simulink model "PI_kalman_discreto"  (R2023b)
settings: Solver=VariableStepAuto  StartTime=0.0  StopTime=200  RelTol=1e-3
undefined symbols (not defined in the file): C_ss, CI, DI, Discrete, dVdt, Ki1, Ki2, Kp1, Kp2, Rn, sigma, step_temp, steptime, Time, Ts, Tsp, Ufeedforward, V0, Vb0, Vmax, Vmin, wd
libraries: slpidlib x2, ctrlSharedLib x1, simulink x1
settings Model: Creator=Maialen  LastModifiedBy=Maialen

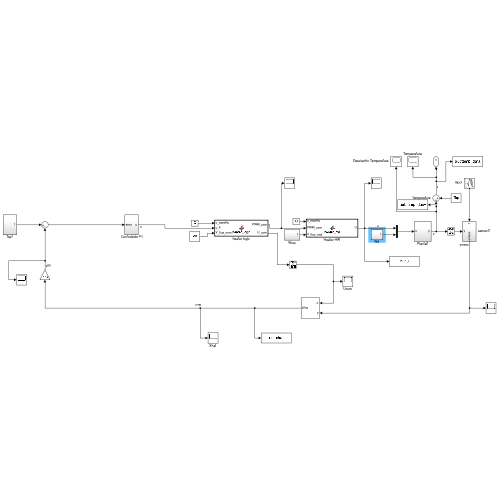
[thumbnail: Simulink's stored preview of the top-level diagram]
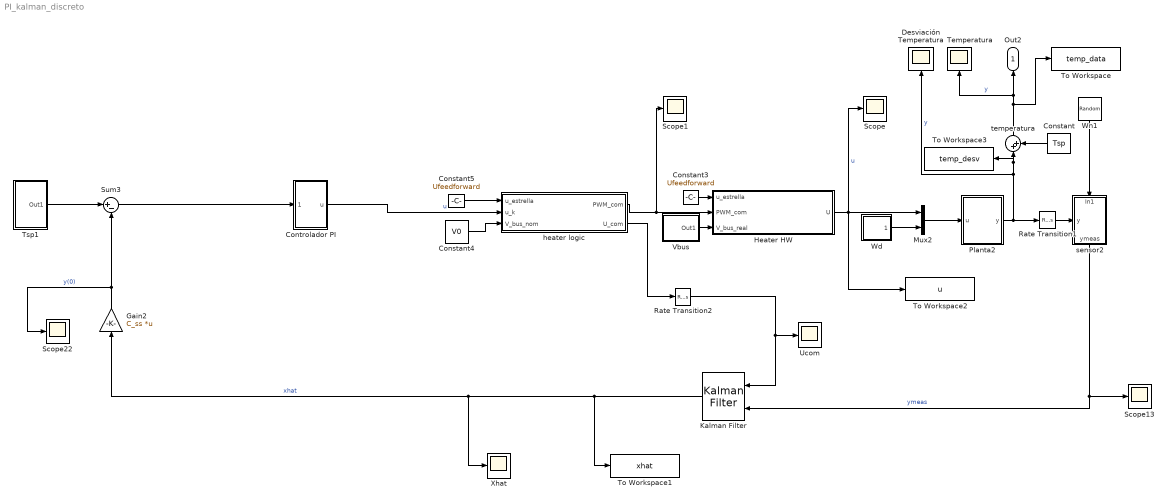
== system PI_kalman_discreto ==
  " Controlador PI" : Subsystem
  Constant : Constant  Value=Tsp  SampleTime=0
  Constant3 : Constant  Value=Ufeedforward  SampleTime=0
  Constant4 : Constant  Value=V0  SampleTime=0
  Constant5 : Constant  Value=Ufeedforward  SampleTime=0
  Desviación Temperatura : Scope
  Gain2 : Gain  Gain=C_ss  Multiplication=Matrix(K*u)
  Heater HW : MATLAB Function  TreatAsAtomicUnit=on
  Kalman Filter : ctrlSharedLib/Kalman Filter  TimeDomain=Discrete-Time  UseCurrentEstimator=on  ModelSource=LTI State-Space Variable  ModelSourceVariable=syskf  A=0.95  B=1  C=1  D=0  NumberOfStates=1  NumberOfInputs=1  NumberOfOutputs=1  InitialEstimateSource=Dialog  X0=0  P0=10  UseK=off  UseGH=off  NumberOfProcessNoiseInputs=1  G=1  TimeInvariantG=on  H=0  TimeInvariantH=on  Q=Qn  TimeInvariantQ=on  R=Rn  TimeInvariantR=on  N=0  TimeInvariantN=on  AddInputPort=on  AddEnablePort=off  OutputEstimatedY=off  OutputP=off  Ts=-1
  Mux2 : Mux  Inputs=2
  Planta2 : Subsystem
  Rate Transition1 : RateTransition  OutPortSampleTime=Ts
  Rate Transition2 : RateTransition  OutPortSampleTime=Ts
  Scope{,1,13,22} (4 alike) : Scope
  Sum3 : Sum  Inputs=|+-
  Temperatura : Scope
  To Workspace : ToWorkspace  VariableName=temp_data  SaveFormat=Timeseries  SampleTime=-1
  To Workspace1 : ToWorkspace  VariableName=xhat  SaveFormat=Timeseries  SampleTime=-1
  To Workspace2 : ToWorkspace  VariableName=u  SaveFormat=Timeseries  SampleTime=-1
  To Workspace3 : ToWorkspace  VariableName=temp_desv  SaveFormat=Timeseries  SampleTime=-1
  Tsp1 : Subsystem
  Ucom : Scope
  Vbus : Subsystem
  Wd : Subsystem
  Wn1 : RandomNumber  Variance=sigma^2  SampleTime=Ts
  Xhat : Scope
  heater logic : MATLAB Function  TreatAsAtomicUnit=on
  sensor2 : Subsystem
      settings: PortSchema="{\"entries\":[{\"content\":{\"sides\":[{\"content\":{\"connectorIds\":[\"In1\"]},\"type\":\"ConnectorPlacement.EquallySpacedRectSide\",\"uuid\":\"87c57665-5a3a-4a29-be31-fc3b8356ea98\"},{\"content\":{\"connectorIds\":[\"Out1\"],\"side\":\"RIGHT\"},\"type\":\"ConnectorPlacement.EquallySpacedRectSide\",\"uuid\":\"3fe956b0-7f9e-4b46-bcb6-e49be4c7e683\"},{\"content\":{\"connectorIds\":[\"In2\"],\"side\":\"TOP\"},\"type\":\"ConnectorPlacement.EquallySpacedRectSide\",\"uuid\":\"3d207620-bc84-4c0d-9751-3dea453ac424\"}]},\"type\":\"ConnectorPlacement.EquallySpacedConnector\",\"uuid\":\"7e1a59fd-e04d-40d6-8549-9ebaaabea5d7\"}],\"packageUris\":[\"http://schema.mathworks.com/mf0/Connector/R2020b\"],\"version\":\"1.0\"}"
  temperatura : Sum  Inputs=|++
  Out2 : Outport
  wires:
  Vbus/1(Out1) -> Heater HW/3(V_bus_real)
  Planta2/1(y) -> Desviación Temperatura/1, To Workspace3/1, temperatura/1, Rate Transition1/1  "y"
  sensor2/1(ymeas) -> Kalman Filter/2, Scope13/1  "ymeas"
  Gain2/1 -> Sum3/2, Scope22/1  "y(0)"
  Wd/1(Out1) -> Mux2/2
  Constant/1 -> temperatura/2
  Constant5/1 -> heater logic/1(u_estrella)
  Wn1/1 -> sensor2/1(In1)
  heater logic/1(PWM_com) -> Heater HW/2(PWM_com), Scope1/1
  Heater HW/1(U) -> Mux2/1, To Workspace2/1, Scope/1  "u"
  Constant4/1 -> heater logic/3(V_bus_nom)
  Constant3/1 -> Heater HW/1(u_estrella)
  Kalman Filter/1 -> To Workspace1/1, Gain2/1, Xhat/1  "xhat"
  Tsp1/1(Out1) -> Sum3/1
  Mux2/1 -> Planta2/1(u)
  temperatura/1 -> To Workspace/1, Temperatura/1, Out2/1  "y"
  heater logic/2(U_com) -> Rate Transition2/1
  Sum3/1 -> " Controlador PI"/1(error)
  " Controlador PI"/1(u) -> heater logic/2(u_k)  "u"
  Rate Transition1/1 -> sensor2/2(y)
  Rate Transition2/1 -> Ucom/1, Kalman Filter/1

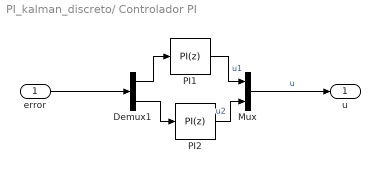
== system PI_kalman_discreto/ Controlador PI ==
  error : Inport
  Demux1 : Demux  Outputs=2
  Mux : Mux  Inputs=2
  "PI1 " : slpidlib/PID Controller  Controller=PI  Form=Parallel  TimeDomain=Discrete-time  UseExternalTs=off  SampleTime=Ts  IntegratorMethod=Forward Euler  FilterMethod=Forward Euler  ControllerParametersSource=internal  P=Kp1  I=Ki1  UseKiTs=off  D=0  N=100  UseFilter=on  TunerSelectOption=Transfer Function Based (PID Tuner App)  InitialConditionSource=internal  InitialConditionForIntegrator=0  InitialConditionForFilter=0  DifferentiatorICPrevScaledInput=0  ExternalReset=none  TrackingMode=off  Kt=1  LimitOutput=off  SatLimitsSource=internal  UpperSaturationLimit=5.7398  LowerSaturationLimit=-5.7398  LinearizeAsGain=on  AntiWindupMode=none  Kb=1  LimitIntegrator=on  UpperIntegratorSaturationLimit=P0  LowerIntegratorSaturationLimit=0  POutMin=[]  POutMax=[]  IOutMin=[]  IOutMax=[]  DOutMin=[]  DOutMax=[]  NOutMin=[]  NOutMax=[]  SumOutMin=[]  SumOutMax=[]  SaturationOutMin=[]  SaturationOutMax=[]  PParamMin=[]  PParamMax=[]  IParamMin=[]  IParamMax=[]  DParamMin=[]  DParamMax=[]  NParamMin=[]  NParamMax=[]  KbParamMin=[]  KbParamMax=[]  KtParamMin=[]  KtParamMax=[]  KbOutMin=[]  KbOutMax=[]  KtOutMin=[]  KtOutMax=[]  IntegratorOutMin=[]  IntegratorOutMax=[]  FilterOutMin=[]  FilterOutMax=[]  SumI1OutMin=[]  SumI1OutMax=[]  SumI2OutMin=[]  SumI2OutMax=[]  SumI3OutMin=[]  SumI3OutMax=[]  SumI4OutMin=[]  SumI4OutMax=[]  SumDOutMin=[]  SumDOutMax=[]  DifferentiatorOutMin=[]  DifferentiatorOutMax=[]  FilterDiffOutCoefMin=[]  FilterDiffOutCoefMax=[]  ReciprocalOutMin=[]  ReciprocalOutMax=[]  SumDenOutMin=[]  SumDenOutMax=[]  SumNumOutMin=[]  SumNumOutMax=[]  DivideOutMin=[]  DivideOutMax=[]  UdiffTsProdOutMin=[]  UdiffTsProdOutMax=[]  NTsProdOutMin=[]  NTsProdOutMax=[]  UintegralTsProdOutMin=[]  UintegralTsProdOutMax=[]  UngainTsProdOutMin=[]  UngainTsProdOutMax=[]  ClampingZeroOutDataTypeStr=Inherit: Inherit via back propagation  ClampingZeroOutMin=[]  ClampingZeroOutMax=[]  FilterDenConstantOutDataTypeStr=Inherit: Inherit via back propagation  FilterDenConstantOutMin=[]  FilterDenConstantOutMax=[]  PCopyOutDataTypeStr=Inherit: Inherit via back propagation  PCopyOutMin=[]  PCopyOutMax=[]  NCopyOutDataTypeStr=Inherit: Inherit via back propagation  NCopyOutMin=[]  NCopyOutMax=[]  IntegratorContinuousStateAttributes=''  IntegratorStateMustResolveToSignalObject=off  IntegratorRTWStateStorageClass=Auto  FilterContinuousStateAttributes=''  FilterStateMustResolveToSignalObject=off  FilterRTWStateStorageClass=Auto  ParallelPVariant=InternalParameters  IdealPVariant=Disabled  IVariant=InternalParameters  DVariant=Disabled  IntegratorVariant=Discrete  SatVariant=Disabled  AWVariant=Passthrough  PCopyVariant=Disabled  TRVariant=Disabled  FdbkBlocksVariant=Forward  IdealPFdbkVariant=Disabled  SatFdbkVariant=Disabled  DerivativeFilterVariant=Disabled  NVariant=Disabled  NCopyVariant=Disabled_SignalSpec  FilterICVariant=Disabled  IntegratorICVariant=InternalICs  ExternalResetVariant=Disabled  TRSumVariant=Passthrough  SumFdbkVariant=Disabled  SumVariant=Sum_PI  TsampFilterVariant=InternalTs  TsampNgainVariant=Passthrough  TsampIntegralVariant=Disabled_SignalSpec  ExternalSaturationOutDataTypeStr=Inherit: Same as second input
  "PI2 " : slpidlib/PID Controller  Controller=PI  Form=Parallel  TimeDomain=Discrete-time  UseExternalTs=off  SampleTime=Ts  IntegratorMethod=Forward Euler  FilterMethod=Forward Euler  ControllerParametersSource=internal  P=Kp2  I=Ki2  UseKiTs=off  D=0  N=100  UseFilter=on  TunerSelectOption=Transfer Function Based (PID Tuner App)  InitialConditionSource=internal  InitialConditionForIntegrator=0  InitialConditionForFilter=0  DifferentiatorICPrevScaledInput=0  ExternalReset=none  TrackingMode=off  Kt=1  LimitOutput=off  SatLimitsSource=internal  UpperSaturationLimit=5.7398  LowerSaturationLimit=-5.7398  LinearizeAsGain=on  AntiWindupMode=none  Kb=1  LimitIntegrator=on  UpperIntegratorSaturationLimit=P0  LowerIntegratorSaturationLimit=0  POutMin=[]  POutMax=[]  IOutMin=[]  IOutMax=[]  DOutMin=[]  DOutMax=[]  NOutMin=[]  NOutMax=[]  SumOutMin=[]  SumOutMax=[]  SaturationOutMin=[]  SaturationOutMax=[]  PParamMin=[]  PParamMax=[]  IParamMin=[]  IParamMax=[]  DParamMin=[]  DParamMax=[]  NParamMin=[]  NParamMax=[]  KbParamMin=[]  KbParamMax=[]  KtParamMin=[]  KtParamMax=[]  KbOutMin=[]  KbOutMax=[]  KtOutMin=[]  KtOutMax=[]  IntegratorOutMin=[]  IntegratorOutMax=[]  FilterOutMin=[]  FilterOutMax=[]  SumI1OutMin=[]  SumI1OutMax=[]  SumI2OutMin=[]  SumI2OutMax=[]  SumI3OutMin=[]  SumI3OutMax=[]  SumI4OutMin=[]  SumI4OutMax=[]  SumDOutMin=[]  SumDOutMax=[]  DifferentiatorOutMin=[]  DifferentiatorOutMax=[]  FilterDiffOutCoefMin=[]  FilterDiffOutCoefMax=[]  ReciprocalOutMin=[]  ReciprocalOutMax=[]  SumDenOutMin=[]  SumDenOutMax=[]  SumNumOutMin=[]  SumNumOutMax=[]  DivideOutMin=[]  DivideOutMax=[]  UdiffTsProdOutMin=[]  UdiffTsProdOutMax=[]  NTsProdOutMin=[]  NTsProdOutMax=[]  UintegralTsProdOutMin=[]  UintegralTsProdOutMax=[]  UngainTsProdOutMin=[]  UngainTsProdOutMax=[]  ClampingZeroOutDataTypeStr=Inherit: Inherit via back propagation  ClampingZeroOutMin=[]  ClampingZeroOutMax=[]  FilterDenConstantOutDataTypeStr=Inherit: Inherit via back propagation  FilterDenConstantOutMin=[]  FilterDenConstantOutMax=[]  PCopyOutDataTypeStr=Inherit: Inherit via back propagation  PCopyOutMin=[]  PCopyOutMax=[]  NCopyOutDataTypeStr=Inherit: Inherit via back propagation  NCopyOutMin=[]  NCopyOutMax=[]  IntegratorContinuousStateAttributes=''  IntegratorStateMustResolveToSignalObject=off  IntegratorRTWStateStorageClass=Auto  FilterContinuousStateAttributes=''  FilterStateMustResolveToSignalObject=off  FilterRTWStateStorageClass=Auto  ParallelPVariant=InternalParameters  IdealPVariant=Disabled  IVariant=InternalParameters  DVariant=Disabled  IntegratorVariant=Discrete  SatVariant=Disabled  AWVariant=Passthrough  PCopyVariant=Disabled  TRVariant=Disabled  FdbkBlocksVariant=Forward  IdealPFdbkVariant=Disabled  SatFdbkVariant=Disabled  DerivativeFilterVariant=Disabled  NVariant=Disabled  NCopyVariant=Disabled_SignalSpec  FilterICVariant=Disabled  IntegratorICVariant=InternalICs  ExternalResetVariant=Disabled  TRSumVariant=Passthrough  SumFdbkVariant=Disabled  SumVariant=Sum_PI  TsampFilterVariant=InternalTs  TsampNgainVariant=Passthrough  TsampIntegralVariant=Disabled_SignalSpec  ExternalSaturationOutDataTypeStr=Inherit: Same as second input
  u : Outport
  wires:
  Mux/1 -> u/1  "u"
  "PI1 "/1 -> Mux/1  "u1"
  error/1 -> Demux1/1
  Demux1/2 -> "PI2 "/1
  "PI2 "/1 -> Mux/2  "u2"
  Demux1/1 -> "PI1 "/1

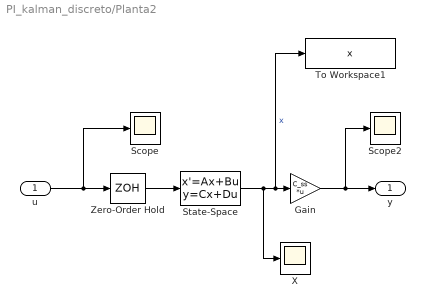
== system PI_kalman_discreto/Planta2 ==
  u : Inport
  Gain : Gain  Gain=C_ss  Multiplication=Matrix(K*u)
  Scope : Scope
  Scope2 : Scope
  State-Space : StateSpace  A=[-28.285755 18.000026 0 0 0 0 0 10.285729 0 0 0 0 0 0 0 0 0 0 0 0 0 0 0 0 0 0 0 0 0 0 0 0 0 0 0 0 0 0;18.000026 -36.000051 18.000026 0 0 0 0 0 0 0 0 0 0 0 0 0 0 0 0 0 0 0 0 0 0 0 0 0 0 0 0 0 0 0 0 0 0 0;0 18.000026 -28.285755 0 0 0 0 0 0 0 0 0 0 0 0 0 0 0 0 0 0 0 0 0 0 0 0 0 0 0 0 0 10.285729 0 0 0 0 0;0 0 0 -28.285755 18.000026 0 10.285729 0 0 0 0 0 0 0 0 0 0 0 0 0 0 0 0 0 0 0 0 0 0 0 0 0 0 0 0 0 0 0;0 0 0 18.000026 -36.000051 18.000026 0 0 0 0 0 0 0 0 0 0 0 0 0 0 0 0 0 0 0 0 0 0 0 0 0 0 0 0 0 0 0 0;0 0 0 0 18.000026 -28.285755 0 0 0 0 0 0 0 0 0 0 0 0 0 0 0 0 0 0 0 0 0 0 0 0 0 0 10.285729 0 0 0 0 0;0 0 0 48 0 0 -48 0 0 0 0 0 0 0 0 0 0 0 0 0 0 0 0 0 0 0 0 0 0 0 0 0 0 0 0 0 0 0;48 0 0 0 0 0 0 -48 0 0 0 0 0 0 0 0 0 0 0 0 0 0 0 0 0 0 0 0 0 0 0 0 0 0 0 0 0 0;0 0 0 0 0 0 0 0 -0.018321982 0.010128496 0 0 0 0 0.0081027967 0 0 0 0 0 0 0 0 0 0 0 0 0 0 0 0 0 0 0 0 0 0 0;0 0 0 0 0 0 0 0 0.010128496 -0.028450675 0.010128496 0 0 0 0 0.0081027967 0 0 0 0 0 0 0 0 0 0 0 0 0 0 0 0 0 0 0 0 0 0;0 0 0 0 0 0 0 0 0 0.010128496 -0.028450922 0.010128496 0 0 0 0 0.0081027967 0 0 0 0 0 0 0 0 0 0 0 0 0 0 0 0 0 0 0 0 0;0 0 0 0 0 0 0 0 0 0 0.010128496 -0.028450922 0.010128496 0 0 0 0 0.0081027967 0 0 0 0 0 0 0 0 0 0 0 0 0 0 0 0 0 0 0 0;0 0 0 0 0 0 0 0 0 0 0 0.010128496 -0.028450675 0.010128496 0 0 0 0 0.0081027967 0 0 0 0 0 0 0 0 0 0 0 0 0 0 0 0 0 0 0;0 0 0 0 0 0 0 0 0 0 0 0 0.010128496 -0.018321982 0 0 0 0 0 0.0081027967 0 0 0 0 0 0 0 0 0 0 0 0 0 0 0 0 0 0;0 0 0 0 0 0 0 0 0.0081027967 0 0 0 0 0 -0.026425101 0.010128496 0 0 0 0 0.0081027967 0 0 0 0 0 0 0 0 0 0 0 0 0 0 0 0 0;0 0 0 0 0 0 0 0 0 0.0081027967 0 0 0 0 0.010128496 -0.036553982 0.010128496 0 0 0 0 0.0081027967 0 0 0 0 0 0 0 0 0 0 0 0 0 0 0 0;0 0 0 0 0 0 0 0 0 0 0.0081027967 0 0 0 0 0.010128496 -0.036554604 0.010128496 0 0 0 0 0.0081027967 0 0 0 0 0 0 0 0 0 0 0 0 0 0 0;0 0 0 0 0 0 0 0 0 0 0 0.0081027967 0 0 0 0 0.010128496 -0.036554604 0.010128496 0 0 0 0 0.0081027967 0 0 0 0 0 0 0 0 0 0 0 0 0 0;0 0 0 0 0 0 0 0 0 0 0 0 0.0081027967 0 0 0 0 0.010128496 -0.036553982 0.010128496 0 0 0 0 0.0081027967 0 0 0 0 0 0 0 0 0 0 0 0 0;0 0 0 0 0 0 0 0 0 0 0 0 0 0.0081027967 0 0 0 0 0.010128496 -0.026425101 0 0 0 0 0 0.0081027967 0 0 0 0 0 0 0 0 0 0 0 0;0 0 0 0 0 0 0 0 0 0 0 0 0 0 0.0081027967 0 0 0 0 0 -0.026425515 0.010128496 0 0 0 0 0.0081027967 0 0 0 0 0 0 0 0 0 0 0;0 0 0 0 0 0 0 0 0 0 0 0 0 0 0 0.0081027967 0 0 0 0 0.010128496 -0.03655478 0.010128496 0 0 0 0 0.0081027967 0 0 0 0 0 0 0 0 0 0;0 0 0 0 0 0 0 0 0 0 0 0 0 0 0 0 0.0081027967 0 0 0 0 0.010128496 -0.089051211 0.010128496 0 0 0 0 0.0081027967 0 0 0 0 0 0 0 0 0.052494331;0 0 0 0 0 0 0 0 0 0 0 0 0 0 0 0 0 0.0081027967 0 0 0 0 0.010128496 -0.089051211 0.010128496 0 0 0 0 0.0081027967 0 0 0 0 0 0 0 0.052494331;0 0 0 0 0 0 0 0 0 0 0 0 0 0 0 0 0 0 0.0081027967 0 0 0 0 0.010128496 -0.03655478 0.010128496 0 0 0 0 0.0081027967 0 0 0 0 0 0 0;0 0 0 0 0 0 0 0 0 0 0 0 0 0 0 0 0 0 0 0.0081027967 0 0 0 0 0.010128496 -0.026425515 0 0 0 0 0 0.0081027967 0 0 0 0 0 0;0 0 0 0 0 0 0 0 0 0 0 0 0 0 0 0 0 0 0 0 0.0081027967 0 0 0 0 0 -0.018322752 0.010128496 0 0 0 0 0 0 0 0 0 0;0 0 0 0 0 0 0 0 0 0 0 0 0 0 0 0 0 0 0 0 0 0.0081027967 0 0 0 0 0.010128496 -0.028451741 0.010128496 0 0 0 0 0 0 0 0 0;0 0 0 0 0 0 0 0 0 0 0 0 0 0 0 0 0 0 0 0 0 0 0.0081027967 0 0 0 0 0.010128496 -0.02845251 0.010128496 0 0 0 0 0 0 0 0;0 0 0 0 0 0 0 0 0 0 0 0 0 0 0 0 0 0 0 0 0 0 0 0.0081027967 0 0 0 0 0.010128496 -0.02845251 0.010128496 0 0 0 0 0 0 0;0 0 0 0 0 0 0 0 0 0 0 0 0 0 0 0 0 0 0 0 0 0 0 0 0.0081027967 0 0 0 0 0.010128496 -0.028451741 0.010128496 0 0 0 0 0 0;0 0 0 0 0 0 0 0 0 0 0 0 0 0 0 0 0 0 0 0 0 0 0 0 0 0.0081027967 0 0 0 0 0.010128496 -0.018322752 0 0 0 0 0 0;0 0 2.2857143 0 0 2.2857143 0 0 0 0 0 0 0 0 0 0 0 0 0 0 0 0 0 0 0 0 0 0 0 0 0 0 -9.3428571 4.7714286 0 0 0 0;0 0 0 0 0 0 0 0 0 0 0 0 0 0 0 0 0 0 0 0 0 0 0 0 0 0 0 0 0 0 0 0 4.7714286 -9.5428571 4.7714286 0 0 0;0 0 0 0 0 0 0 0 0 0 0 0 0 0 0 0 0 0 0 0 0 0 0 0 0 0 0 0 0 0 0 0 0 4.7714286 -10.228571 5.4571429 0 0;0 0 0 0 0 0 0 0 0 0 0 0 0 0 0 0 0 0 0 0 0 0 0 0 0 0 0 0 0 0 0 0 0 0 5.4571429 -11.819048 6.3619048 0;0 0 0 0 0 0 0 0 0 0 0 0 0 0 0 0 0 0 0 0 0 0 0 0 0 0 0 0 0 0 0 0 0 0 0 6.3619048 -11.819048 5.4571429;0 0 0 0 0 0 0 0 0 0 0 0 0 0 0 0 0 0 0 0 0 0 2.6457143 2.6457143 0 0 0 0 0 0 0 0 0 0 0 0 5.4571429 -10.748571]  B=[0 0 0;0 0 0;0 0 0;0 0 0;0 0 0;0 0 0;0 0 0;0 0 0;0 0 0.00078735198;0 0 0.00078735198;0 0 0.00078735198;0 0 0.00078735198;0 0 0.00078735198;0 0 0.00078735198;0 0 0.00078735198;0 0 0.00078735198;0 0 0.00078735198;0 0 0.00078735198;0 0 0.00078735198;0 0 0.00078735198;0 0 0.00078735198;0 0 0.00078735198;0.0094482237 0 0.00078735198;0.0094482237 0 0.00078735198;0 0 0.00078735198;0 0 0.00078735198;0 0 0.00078735198;0 0 0.00078735198;0 0 0.00078735198;0 0 0.00078735198;0 0 0.00078735198;0 0 0.00078735198;0 0 0;0 0.95238095 0;0 0 0;0 0 0;0 0 0;0 0 0]  C=CI  D=DI  InitialCondition=0
  To Workspace1 : ToWorkspace  VariableName=x  SaveFormat=Timeseries  SampleTime=-1
  X : Scope
  Zero-Order Hold : ZeroOrderHold  SampleTime=Ts
  y : Outport
  wires:
  u/1 -> Scope/1, Zero-Order Hold/1
  Gain/1 -> Scope2/1, y/1
  State-Space/1 -> X/1, To Workspace1/1, Gain/1  "x"
  Zero-Order Hold/1 -> State-Space/1

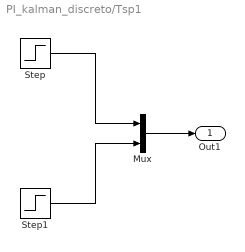
== system PI_kalman_discreto/Tsp1 ==
  Mux : Mux  Inputs=2
  Step : Step  Time=steptime  After=step_temp  SampleTime=0
  Step1 : Step  Time=steptime  After=step_temp  SampleTime=0
  Out1 : Outport
  wires:
  Mux/1 -> Out1/1
  Step1/1 -> Mux/2
  Step/1 -> Mux/1

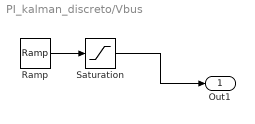
== system PI_kalman_discreto/Vbus ==
  Ramp : simulink/Sources/Ramp  slope=dVdt  start=steptime  InitialOutput=Vb0
  Saturation : Saturate  UpperLimit=Vmax  LowerLimit=Vmin
  Out1 : Outport
  wires:
  Ramp/1 -> Saturation/1
  Saturation/1 -> Out1/1

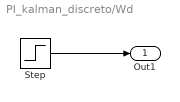
== system PI_kalman_discreto/Wd ==
  Step : Step  Time=steptime  After=wd  SampleTime=0
  Out1 : Outport
  wires:
  Step/1 -> Out1/1

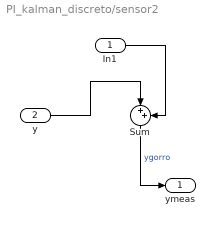
== system PI_kalman_discreto/sensor2 ==
  In1 : Inport
  y : Inport  Port=2
  Sum : Sum  Inputs=|++
  ymeas : Outport
  wires:
  In1/1 -> Sum/2
  y/1 -> Sum/1
  Sum/1 -> ymeas/1  "ygorro"

== matlab function PI_kalman_discreto/Heater HW ==
  data: u_estrella input; PWM_com input; U output; V_bus_real input
function U = heater_hw(u_estrella, PWM_com, V_bus_real)
    R_real = [156.8; 156.8];
    
    % Potencia real entregada a la planta
    P_max_real = (V_bus_real^2) ./ R_real;
    U= PWM_com .* P_max_real - u_estrella;
end

== matlab function PI_kalman_discreto/heater logic ==
  data: u_estrella input; u_k input; PWM_com output; V_bus_nom input; U_com output
function [PWM_com, U_com] = heater_logic(u_estrella, u_k, V_bus_nom)
    R0 = [156.8; 156.8];
    
    % Potencia máxima disponible
    P_max = (V_bus_nom^2) ./ R0;
    
    % Potencia absoluta demandada = feedforward + corrección LQR (desviación)
    P_demanda = u_estrella + u_k;
    
    % Saturación física
    P_limitada = max(0, min(P_max, P_demanda));
    
    % PWM lineal
    PWM_com = P_limitada ./ P_max;
    
    % Anti-windup: congela integrador si satura
    sat_arriba = P_demanda >= P_max;
    sat_abajo  = P_demanda <= 0;
    stop_int   = double(~(sat_arriba | sat_abajo));
    
    % Potencia comandada (para el Kalman)
    U_com = P_limitada - u_estrella;
end
